simulink model "cv04"  (R2024b)
settings: Solver=VariableStepAuto  StartTime=0.0  StopTime=10000  RelTol=1e-3
undefined symbols (not defined in the file): m, n
libraries: sldelib x1
settings Model: Creator=baron  LastModifiedBy=baron

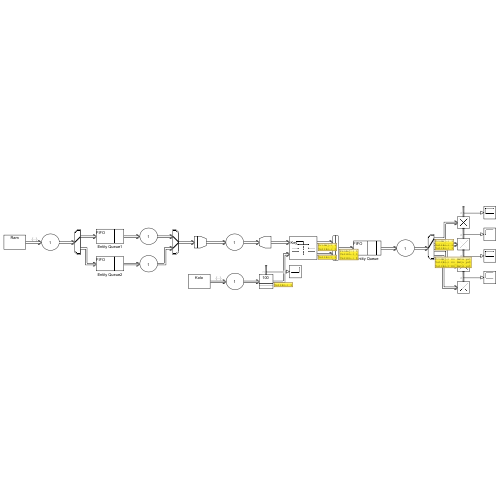
[thumbnail: Simulink's stored preview of the top-level diagram]
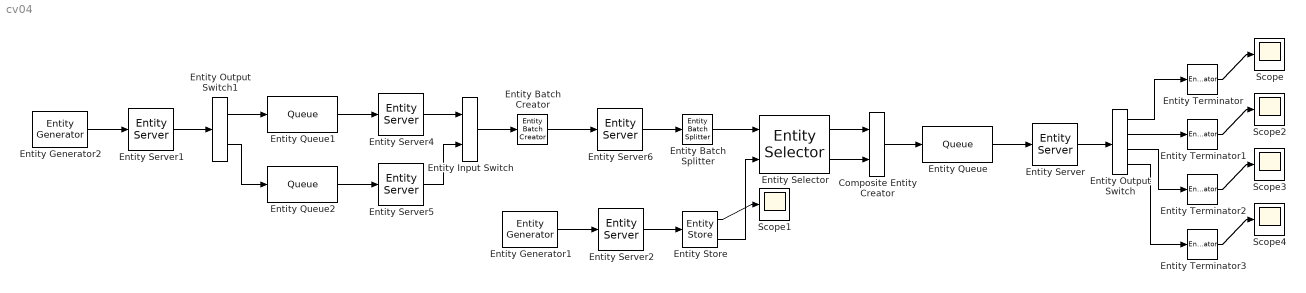
== system cv04 ==
  Composite Entity Creator : CompositeEntityCreator  InputPortMessageModes=m,m  OutputPortMessageModes=m  EntityTypeName=Combined
      settings: InputPortMap=u0,u1
  Entity Input Switch : EntityInputSwitch  InputPortMessageModes=m,m  OutputPortMessageModes=m
  Entity Output Switch : EntityOutputSwitch  InputPortMessageModes=m  OutputPortMessageModes=m,m,m,m  NumberOutputPorts=4  SwitchingCriterion=From attribute  SwitchAttributeName=E1.Prodejny
      settings: OutputPortMap=o0,o1,o2,o3
  Entity Output Switch1 : EntityOutputSwitch  InputPortMessageModes=m  OutputPortMessageModes=m,m  SwitchingCriterion=From attribute  SwitchAttributeName=Velikost
  Entity Batch Creator : EntityBatchCreator  InputPortMessageModes=m  OutputPortMessageModes=m  NumberOfEntitiesInBatch=10
      settings: OutputPortMap=o4
  Entity Batch Splitter : EntityBatchSplitter  InputPortMessageModes=m  OutputPortMessageModes=m
      settings: OutputPortMap=o4
  Entity Generator1 : EntityGenerator  OutputPortMessageModes=m  Period=5  AttributeName=Velikost  EntityType=Structured  EntityTypeName=Kolo
  Entity Generator2 : EntityGenerator  OutputPortMessageModes=m  TimeSource=MATLAB action  IntergenerationTimeAction=|  AttributeName=Prodejny|Velikost  AttributeInitialValue=1|1  EntityType=Structured  EntityTypeName=Ram
      | persistent rngInit;
      | if isempty(rngInit)
      |     seed = 12345;
      |     rng(seed);
      |     rngInit = true;
      | end
      | 
      | % Pattern: Uniform distribution
      | % m: Minimum, M: Maximum
      | m = 0; M = 10;
      | dt = m + (M - m) * rand;
  Entity Queue : Queue  InputPortMessageModes=m  OutputPortMessageModes=m
  Entity Queue1 : Queue  InputPortMessageModes=m  OutputPortMessageModes=m
  Entity Queue2 : Queue  InputPortMessageModes=m  OutputPortMessageModes=m
  Entity Selector : sldelib/Entity Selector  mNumberOfStreams=1  mKeyEntityAttributeName={'Velikost'}  mEntityAttributeName={'Velikost'}  mMatchingNumberSource=Dialog  mNumberOfMatches=1  mNumberOfMatchesAttribute=Name  mNumEntitiesDepOpt=off  mNumEntitiesInBlockOpt=off  mNumEntitiesExtractedOpt=off
  Entity Server : EntityServer  InputPortMessageModes=m  OutputPortMessageModes=m  Capacity=1
  Entity Server1 : EntityServer  InputPortMessageModes=m  OutputPortMessageModes=m  Capacity=1  EntryAction=|
      | entity.Prodejny = randi([1,4]);
      | entity.Velikost = randi([1,2]);
  Entity Server2 : EntityServer  InputPortMessageModes=m  OutputPortMessageModes=m  Capacity=1  EntryAction=entity.Velikost = randi([1,2]);
  Entity Server4 : EntityServer  InputPortMessageModes=m  OutputPortMessageModes=m  Capacity=1
  Entity Server5 : EntityServer  InputPortMessageModes=m  OutputPortMessageModes=m  Capacity=1  ServiceTimeValue=2
  Entity Server6 : EntityServer  InputPortMessageModes=m  OutputPortMessageModes=m  Capacity=1  ServiceTimeValue=200
  Entity Store : EntityStore  InputPortMessageModes=m  OutputPortMessageModes=n,m  Capacity=100  NumberEntitiesInBlock=on
      settings: OutputPortMap=o1,o4
  Entity Terminator{,1..3} (4 alike) : EntityTerminator  InputPortMessageModes=m  NumberEntitiesArrived=on
      settings: OutputPortMap=o0
  Scope{,1..4} (5 alike) : Scope
  wires:
  Entity Batch Splitter/1 -> Entity Selector/1
  Entity Queue1/1 -> Entity Server4/1
  Entity Server2/1 -> Entity Store/1
  Entity Server4/1 -> Entity Input Switch/1
  Entity Output Switch1/2 -> Entity Queue2/1
  Entity Output Switch1/1 -> Entity Queue1/1
  Entity Server1/1 -> Entity Output Switch1/1
  Entity Generator2/1 -> Entity Server1/1
  Entity Queue2/1 -> Entity Server5/1
  Entity Input Switch/1 -> Entity Batch Creator/1
  Entity Server5/1 -> Entity Input Switch/2
  Entity Batch Creator/1 -> Entity Server6/1
  Entity Selector/1 -> Composite Entity Creator/1
  Entity Generator1/1 -> Entity Server2/1
  Entity Server6/1 -> Entity Batch Splitter/1
  Entity Store/1 -> Scope1/1
  Entity Store/2 -> Entity Selector/2
  Entity Selector/2 -> Composite Entity Creator/2
  Composite Entity Creator/1 -> Entity Queue/1
  Entity Queue/1 -> Entity Server/1
  Entity Server/1 -> Entity Output Switch/1
  Entity Output Switch/1 -> Entity Terminator/1
  Entity Output Switch/2 -> Entity Terminator1/1
  Entity Output Switch/3 -> Entity Terminator2/1
  Entity Output Switch/4 -> Entity Terminator3/1
  Entity Terminator/1 -> Scope/1
  Entity Terminator2/1 -> Scope3/1
  Entity Terminator1/1 -> Scope2/1
  Entity Terminator3/1 -> Scope4/1
